simulink model "WS1simulink"  (R2023a)
settings: Solver=VariableStepAuto  StartTime=0.0  StopTime=1  RelTol=1e-3
values from neighbouring files (symbols this model uses):
  D = 3.5077E-6    (= 3.5077e-06)    [setupModelParametersWs1.m]
  J = 3.2284E-6    (= 3.2284e-06)    [setupModelParametersWs1.m]
  K = 0.0274    [setupModelParametersWs1.m]
  L = 5.5E-6    (= 5.5e-06)    [setupModelParametersWs1.m]
  R = 4    [setupModelParametersWs1.m]
settings Model: Creator=socks  LastModifiedBy=socks

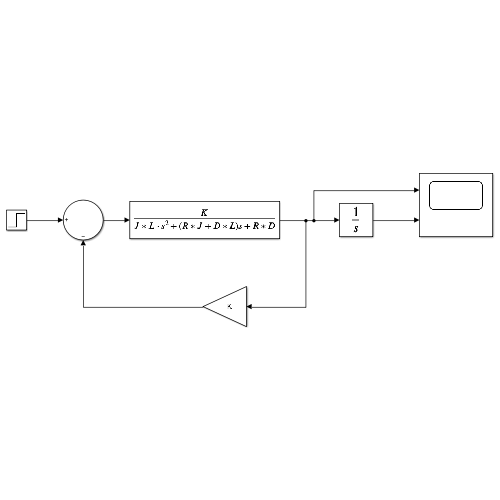
[thumbnail: Simulink's stored preview of the top-level diagram]
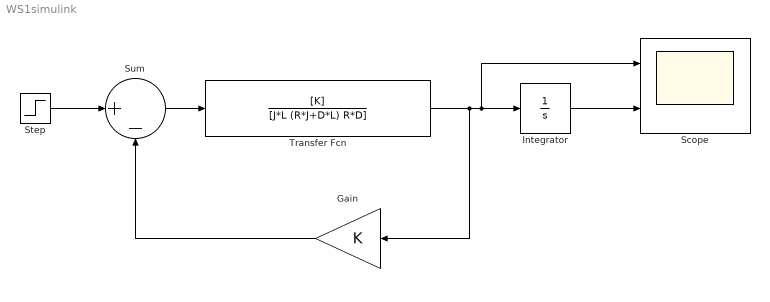
== system WS1simulink ==
  Gain : Gain  Gain=K
  Integrator : Integrator
  Scope : Scope  NumInputPorts=2
  Step : Step  Time=0  SampleTime=0
  Sum : Sum  Inputs=|+-
  Transfer Fcn : TransferFcn  Numerator=[K]  Denominator=[J*L (R*J+D*L) R*D]
  wires:
  Gain/1 -> Sum/2
  Sum/1 -> Transfer Fcn/1
  Transfer Fcn/1 -> Gain/1, Scope/1, Integrator/1
  Step/1 -> Sum/1
  Integrator/1 -> Scope/2
